simulink model "model"  (R2020b)
settings: Solver=VariableStepAuto  StartTime=0.0  StopTime=10.0  RelTol=1e-3
model workspace (MAT data in the model file):
  ParamCopy4 = Simulink.Parameter
  ParamCopy4.DataType = 'auto'
  ParamCopy4.Dimensions = [0 0]
  ParamCopy5 = Simulink.Parameter
  ParamCopy5.DataType = 'auto'
  ParamCopy5.Dimensions = [0 0]
  b = Simulink.Parameter
  b.Value = 3.5077e-06
  b.DataType = 'auto'
  b.Dimensions = [1 1]
  j = Simulink.Parameter
  j.Value = 3.2284e-06
  j.DataType = 'auto'
  j.Dimensions = [1 1]
  k = Simulink.Parameter
  k.Value = 0.0274
  k.DataType = 'auto'
  k.Dimensions = [1 1]
  l = Simulink.Parameter
  l.Value = 2.75e-06
  l.DataType = 'auto'
  l.Dimensions = [1 1]
  r = Simulink.Parameter
  r.Value = 4
  r.DataType = 'auto'
  r.Dimensions = [1 1]
settings Model: Creator=SAGAR  LastModifiedBy=SAGAR

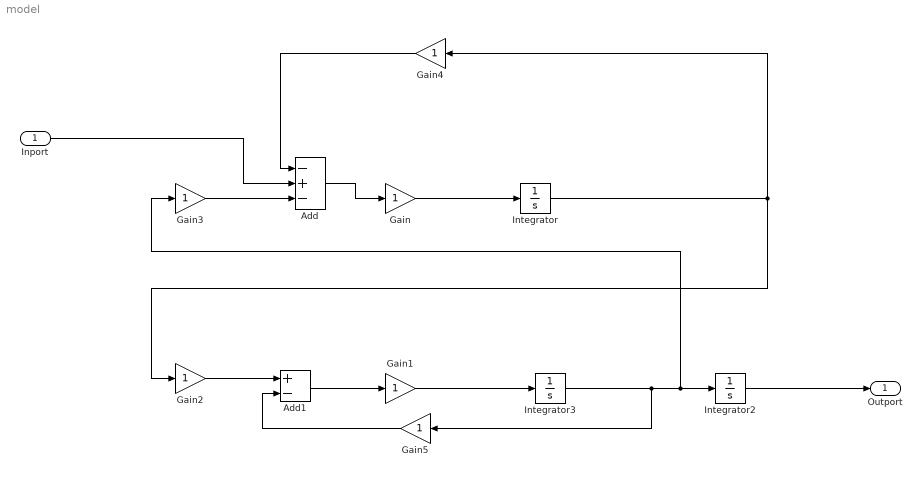
== system model ==
  Inport : Inport
  Add : Sum  Inputs=-+-
  Add1 : Sum  Inputs=+-
  Gain{,1..5} (6 alike) : Gain
  Integrator : Integrator
  Integrator2 : Integrator
  Integrator3 : Integrator
  Outport : Outport
  wires:
  Gain2/1 -> Add1/1
  Add1/1 -> Gain1/1
  Gain3/1 -> Add/3
  Add/1 -> Gain/1
  Gain4/1 -> Add/1
  Gain/1 -> Integrator/1
  Gain1/1 -> Integrator3/1
  Integrator3/1 -> Gain5/1, Gain3/1, Integrator2/1
  Integrator/1 -> Gain4/1, Gain2/1
  Inport/1 -> Add/2
  Gain5/1 -> Add1/2
  Integrator2/1 -> Outport/1
